simulink model "fsk"  (Simulink 10.3)
settings: Solver=VariableStepAuto  StartTime=0.0  StopTime=0.02  RelTol=1e-3
values from neighbouring files (symbols this model uses):
  Data_BitRate = 200    [main.m]
  High_Freq = Low_Freq * 5    (= 5000)    [main.m]
  Low_Freq = 1000    [main.m]
  Sampling_Freq = 1000 * High_Freq    (= 5000000)    [main.m]
  Sin_Signal = sin(Sin_Signal_Time_Step)    [main.m]
  Sin_Signal_Index = 0:Sin_Signal_Samples    [main.m]
settings Model: Creator=alireza  LastModifiedBy=alireza
settings SolverCC: AlgebraicLoopSolver=Auto
settings DataIOCC: SaveFormat=Dataset  SignalLoggingSaveFormat=Dataset  ReturnWorkspaceOutputs=on
settings OptimizationCC: ExpressionDepthLimit=128  LifeSpan=auto
settings DebuggingCC: UnderspecifiedInitializationDetection=Simplified  MergeDetectMultiDrivingBlocksExec=error  FcnCallInpInsideContextMsg=error  StateNameClashWarn=none  SFUnexpectedBacktrackingDiag=error  SFNoUnconditionalDefaultTransitionDiag=error  SFExecutionAtInitializationDiag=warning  SFMachineParentedDataDiag=error  ArithmeticOperatorsInVariantConditions=error
settings HardwareCC: ProdBitPerPointer=64  ProdBitPerSizeT=64  ProdBitPerPtrDiffT=64  ProdLargestAtomicFloat=Float  ProdIntDivRoundTo=Zero  ProdEndianess=LittleEndian  ProdWordSize=64  ProdHWDeviceType=Intel->x86-64 (Windows64)
settings ModelReferenceCC: PropagateSignalLabelsOutOfModel=on
settings SFSimCC: SimUseLocalCustomCode=on  CustomCodeUndefinedFunction=FilterOut
settings RTWCC: RTWUseLocalCustomCode=on
settings CodeAppCC: StateflowObjectComments=off
settings GRTTargetCC: TargetLangStandard=C99 (ISO)  CombineOutputUpdateFcns=on  GRTInterface=off
settings ConfigComp: CovMetricSettings=dwe  CovSaveCumulativeToWorkspaceVar=off  CovSaveSingleToWorkspaceVar=off  CovExternalEMLEnable=on

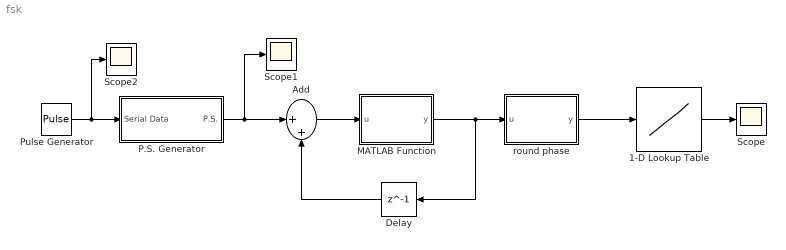
== system fsk ==
  1-D Lookup Table : Lookup_n-D  NumberOfTableDimensions=1  BreakpointsForDimension1=Sin_Signal_Index  Table=Sin_Signal  InternalRulePriority=Speed  RndMeth=Simplest  InputSameDT=on
  Add : Sum  Inputs=|++
  Delay : Delay  DelayLength=1  InitialCondition=0  SampleTime=1/Sampling_Freq
  MATLAB Function : MATLAB Function  TreatAsAtomicUnit=on
  P.S. Generator : Subsystem
  Pulse Generator : DiscretePulseGenerator  PulseType=Time based  Period=(1*2)/Data_BitRate  PulseWidth=50
  Scope : Scope
  Scope1 : Scope
  Scope2 : Scope
  round phase : MATLAB Function  TreatAsAtomicUnit=on
  wires:
  P.S. Generator/1(P.S.) -> Add/1, Scope1/1
  Add/1 -> MATLAB Function/1(u)
  MATLAB Function/1(y) -> round phase/1(u), Delay/1
  Delay/1 -> Add/2
  round phase/1(y) -> 1-D Lookup Table/1
  1-D Lookup Table/1 -> Scope/1
  Pulse Generator/1 -> Scope2/1, P.S. Generator/1(Serial Data)

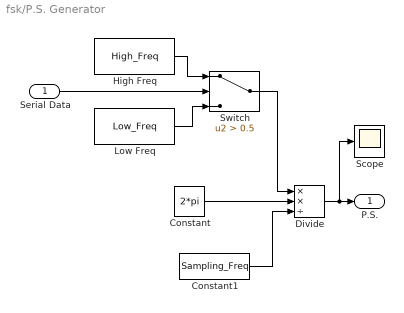
== system fsk/P.S. Generator ==
  Serial Data : Inport
  Constant : Constant  Value=2*pi
  Constant1 : Constant  Value=Sampling_Freq
  Divide : Product  Inputs=**/
  High Freq : Constant  Value=High_Freq
  Low Freq : Constant  Value=Low_Freq
  Scope : Scope
  Switch : Switch  Criteria=u2 > Threshold  Threshold=0.5
  P.S. : Outport
  wires:
  Constant/1 -> Divide/2
  Constant1/1 -> Divide/3
  Divide/1 -> Scope/1, P.S./1
  Switch/1 -> Divide/1
  High Freq/1 -> Switch/1
  Low Freq/1 -> Switch/3
  Serial Data/1 -> Switch/2

== matlab function round phase ==
  data: u input double; y output double
function y = phase2ind(u)
    y = round(u * 1800 / (2 * pi));

== matlab function MATLAB Function ==
  data: u input double; y output double
function y = Current_Phi(u)
    y = rem(u,2*pi);
